simulink model "Pgenerationsimulink_chapter5_method2"  (R2023a)
settings: Solver=VariableStepAuto  StartTime=0.0  StopTime=10.0  RelTol=1e-3  EnableMultiTasking=on
values from neighbouring files (symbols this model uses):
  Cz = [k0 c0 -k0 -c0 1]    [Chapter5_method2.m]
libraries: cstblocks x4
settings Model: Creator=Administrator  LastModifiedBy=senameo
settings SolverCC: AlgebraicLoopSolver=TrustRegion
settings DataIOCC: LimitDataPoints=on  ReturnWorkspaceOutputs=off
settings OptimizationCC: LifeSpan=inf
settings DebuggingCC: UnconnectedInputMsg=warning  UnconnectedOutputMsg=warning  UnconnectedLineMsg=warning  AllowSymbolicDim=off  SFUnexpectedBacktrackingDiag=warning  SFNoUnconditionalDefaultTransitionDiag=warning  SFExecutionAtInitializationDiag=none  ArithmeticOperatorsInVariantConditions=warning
settings ModelReferenceCC: EnableRefExpFcnMdlSchedulingChecks=on  PropagateSignalLabelsOutOfModel=off
settings SFSimCC: SimUseLocalCustomCode=off  CustomCodeUndefinedFunction=UseInterfaceOnly
settings RTWCC: RTWUseLocalCustomCode=off  DLArmComputeVersion=19.05
settings CodeAppCC: StateflowObjectComments=on
settings GRTTargetCC: TargetLangStandard=C89/C90 (ANSI)
settings ConfigComp: CovMetricSettings=dw  CovSaveCumulativeToWorkspaceVar=on  CovSaveSingleToWorkspaceVar=on  CovExternalEMLEnable=off

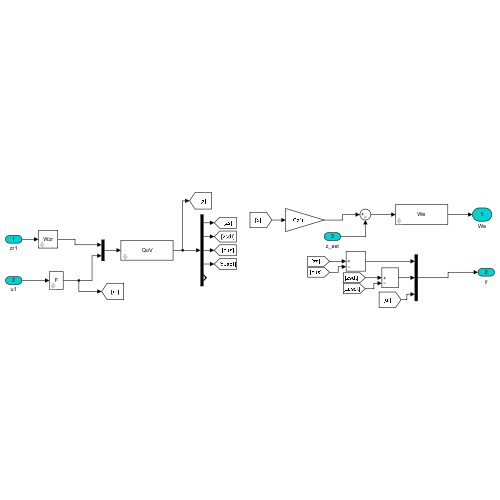
[thumbnail: Simulink's stored preview of the top-level diagram]
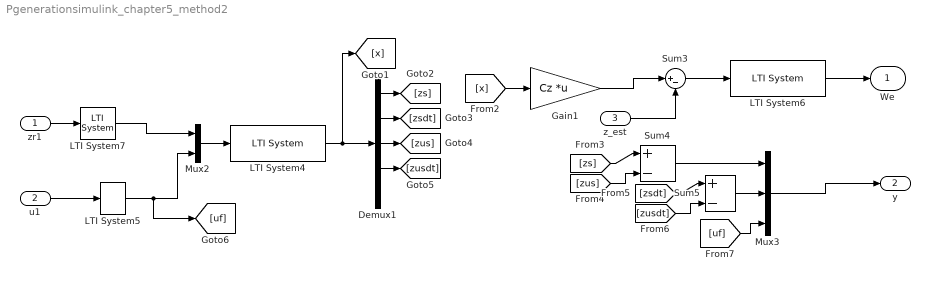
== system Pgenerationsimulink_chapter5_method2 ==
  zr1 : Inport  PortDimensions=1
  u1 : Inport  Port=2  PortDimensions=1
  z_est : Inport  Port=3  PortDimensions=1
  Demux1 : Demux  Outputs=5
  Gain1 : Gain  Gain=Cz  Multiplication=Matrix(K*u)
  LTI System4 : cstblocks/LTI System  sys=QoV  IC=[]
  LTI System5 : cstblocks/LTI System  sys=F  IC=[]
  LTI System6 : cstblocks/LTI System  sys=We  IC=[]
  LTI System7 : cstblocks/LTI System  sys=Wzr  IC=[]
  Mux2 : Mux  Inputs=2
  Mux3 : Mux  Inputs=3
  Sum3 : Sum  Inputs=|+-
  Sum4 : Sum  Inputs=|+-
  Sum5 : Sum  Inputs=|+-
  We : Outport  PortDimensions=1  VectorParamsAs1DForOutWhenUnconnected=off
  y : Outport  Port=2  PortDimensions=3  VectorParamsAs1DForOutWhenUnconnected=off
  wires:
  LTI System5/1 -> [uf], Mux2/2
  u1/1 -> LTI System5/1
  LTI System7/1 -> Mux2/1
  zr1/1 -> LTI System7/1
  Mux2/1 -> LTI System4/1
  LTI System4/1 -> [x], Demux1/1
  Demux1/1 -> [zs]
  Demux1/2 -> [zsdt]
  Demux1/3 -> [zus]
  Demux1/4 -> [zusdt]
  Sum3/1 -> LTI System6/1
  Gain1/1 -> Sum3/1
  LTI System6/1 -> We/1
  z_est/1 -> Sum3/2
  [x] -> Gain1/1
  Sum5/1 -> Mux3/2
  Sum4/1 -> Mux3/1
  Mux3/1 -> y/1
  [zs] -> Sum4/1
  [zus] -> Sum4/2
  [zsdt] -> Sum5/1
  [zusdt] -> Sum5/2
  [uf] -> Mux3/3
